simulink model "sensor_simulation"  (R2018a)
settings: Solver=VariableStepAuto  StartTime=0.0  StopTime=10.0  RelTol=1e-3
libraries: simulink x16
(part 1 of 2)
settings Model: Creator=vsbdh  LastModifiedBy=vsbdh

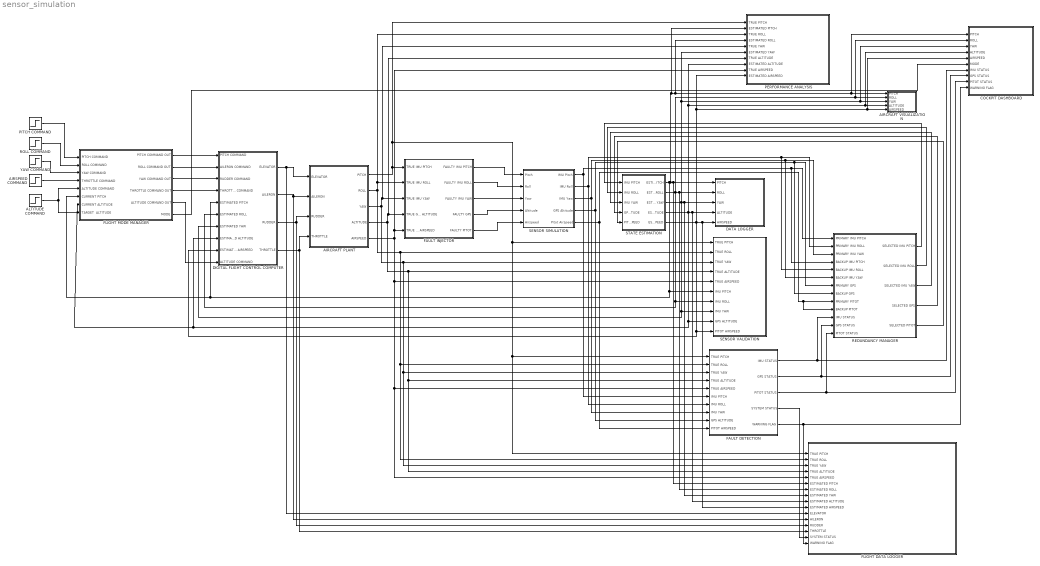
== system sensor_simulation ==
  " SENSOR VALIDATION" : Subsystem
  AIRCRAFT PLANT : Subsystem
  AIRCRAFT VISUALIZATION : Subsystem
  AIRSPEED COMMAND : Step  Time=0  SampleTime=0
  ALTITUDE COMMAND : Step  Time=2  After=1000  SampleTime=0
  COCKPIT DASHBOARD : Subsystem
  DATA LOGGER : Subsystem
  DIGITAL FLIGHT CONTROL COMPUTER : Subsystem
  FAULT DETECTION : Subsystem
  "FAULT INJECTOR " : Subsystem
  FLIGHT DATA LOGGER : Subsystem
  FLIGHT MODE MANAGER : Subsystem
  PERFORMANCE ANALYSIS : Subsystem
  PITCH COMMAND : Step  Time=0  SampleTime=0
  REDUNDANCY MANAGER : Subsystem
  ROLL COMMAND : Step  Time=0  SampleTime=0
  SENSOR SIMULATION : Subsystem
  STATE ESTIMATION : Subsystem
  YAW COMMAND : Step  Time=0  SampleTime=0
  wires:
  AIRCRAFT PLANT/1(PITCH) -> "FAULT INJECTOR "/1(TRUE IMU PITCH), PERFORMANCE ANALYSIS/1(TRUE PITCH), FLIGHT DATA LOGGER/1(TRUE PITCH), FAULT DETECTION/1(TRUE PITCH), " SENSOR VALIDATION"/1(TRUE PITCH)
  AIRCRAFT PLANT/2(ROLL) -> PERFORMANCE ANALYSIS/3(TRUE ROLL), "FAULT INJECTOR "/2(TRUE IMU ROLL), " SENSOR VALIDATION"/2(TRUE ROLL), FAULT DETECTION/2(TRUE ROLL), FLIGHT DATA LOGGER/2(TRUE ROLL)
  AIRCRAFT PLANT/3(YAW) -> PERFORMANCE ANALYSIS/5(TRUE YAW), "FAULT INJECTOR "/3(TRUE IMU YAW), FLIGHT DATA LOGGER/3(TRUE YAW), FAULT DETECTION/3(TRUE YAW), " SENSOR VALIDATION"/3(TRUE YAW)
  AIRCRAFT PLANT/4(ALTITUDE) -> FAULT DETECTION/4(TRUE ALTITUDE), FLIGHT DATA LOGGER/4(TRUE ALTITUDE), " SENSOR VALIDATION"/4(TRUE ALTITUDE), PERFORMANCE ANALYSIS/7(TRUE ALTITUDE), "FAULT INJECTOR "/4(TRUE GPS ALTITUDE)
  AIRCRAFT PLANT/5(AIRSPEED) -> PERFORMANCE ANALYSIS/9(TRUE AIRSPEED), "FAULT INJECTOR "/5(TRUE PITOT AIRSPEED), " SENSOR VALIDATION"/5(TRUE AIRSPEED), FAULT DETECTION/5(TRUE AIRSPEED), FLIGHT DATA LOGGER/5(TRUE AIRSPEED)
  SENSOR SIMULATION/1(IMU Pitch) -> FAULT DETECTION/6(IMU PITCH), REDUNDANCY MANAGER/1(PRIMARY IMU PITCH), REDUNDANCY MANAGER/4(BACKUP IMU PITCH)
  SENSOR SIMULATION/2(IMU Roll) -> FAULT DETECTION/7(IMU ROLL), REDUNDANCY MANAGER/5(BACKUP IMU ROLL), REDUNDANCY MANAGER/2(PRIMARY IMU ROLL)
  SENSOR SIMULATION/3(IMU Yaw) -> FAULT DETECTION/8(IMU YAW), REDUNDANCY MANAGER/6(BACKUP IMU YAW), REDUNDANCY MANAGER/3(PRIMARY IMU YAW)
  SENSOR SIMULATION/4(GPS Altitude) -> FAULT DETECTION/9(GPS ALTITUDE), REDUNDANCY MANAGER/8(BACKUP GPS), REDUNDANCY MANAGER/7(PRIMARY GPS)
  SENSOR SIMULATION/5(Pitot Airspeed) -> FAULT DETECTION/10(PITOT AIRSPEED), REDUNDANCY MANAGER/10(BACKUP PITOT), REDUNDANCY MANAGER/9(PRIMARY PITOT)
  STATE ESTIMATION/1(ESTIMATED PITCH) -> PERFORMANCE ANALYSIS/2(ESTIMATED PITCH), PERFORMANCE ANALYSIS/4(ESTIMATED ROLL), COCKPIT DASHBOARD/1(PITCH), AIRCRAFT VISUALIZATION/1(PITCH), DATA LOGGER/1(PITCH), FLIGHT DATA LOGGER/6(ESTIMATED PITCH), FLIGHT MODE MANAGER/6(CURRENT PITCH), DIGITAL FLIGHT CONTROL COMPUTER/5(ESTIMATED PITCH), " SENSOR VALIDATION"/6(IMU PITCH)
  STATE ESTIMATION/2(ESTIMATED ROLL) -> DIGITAL FLIGHT CONTROL COMPUTER/6(ESTIMATED ROLL), " SENSOR VALIDATION"/7(IMU ROLL), COCKPIT DASHBOARD/2(ROLL), AIRCRAFT VISUALIZATION/2(ROLL), FLIGHT DATA LOGGER/7(ESTIMATED ROLL), DATA LOGGER/2(ROLL)
  STATE ESTIMATION/3(ESTIMATED YAW) -> DIGITAL FLIGHT CONTROL COMPUTER/7(ESTIMATED YAW), " SENSOR VALIDATION"/8(IMU YAW), PERFORMANCE ANALYSIS/6(ESTIMATED YAW), COCKPIT DASHBOARD/3(YAW), AIRCRAFT VISUALIZATION/3(YAW), FLIGHT DATA LOGGER/8(ESTIMATED YAW), DATA LOGGER/3(YAW)
  STATE ESTIMATION/4(ESTIMATED ALTITUDE) -> PERFORMANCE ANALYSIS/8(ESTIMATED ALTITUDE), COCKPIT DASHBOARD/4(ALTITUDE), AIRCRAFT VISUALIZATION/4(ALTITUDE), FLIGHT DATA LOGGER/9(ESTIMATED ALTITUDE), DATA LOGGER/4(ALTITUDE), DIGITAL FLIGHT CONTROL COMPUTER/8(ESTIMATED ALTITUDE), FLIGHT MODE MANAGER/7(CURRENT ALTITUDE), " SENSOR VALIDATION"/9(GPS ALTITUDE)
  STATE ESTIMATION/5(ESTIMATED AIRSPEED) -> PERFORMANCE ANALYSIS/10(ESTIMATED AIRSPEED), COCKPIT DASHBOARD/5(AIRSPEED), AIRCRAFT VISUALIZATION/5(AIRSPEED), FLIGHT DATA LOGGER/10(ESTIMATED AIRSPEED), DATA LOGGER/5(AIRSPEED), DIGITAL FLIGHT CONTROL COMPUTER/9(ESTIMATED AIRSPEED), " SENSOR VALIDATION"/10(PITOT AIRSPEED)
  DIGITAL FLIGHT CONTROL COMPUTER/1(ELEVATOR) -> FLIGHT DATA LOGGER/11(ELEVATOR), AIRCRAFT PLANT/1(ELEVATOR)
  DIGITAL FLIGHT CONTROL COMPUTER/2(AILERON) -> FLIGHT DATA LOGGER/12(AILERON), AIRCRAFT PLANT/2(AILERON)
  DIGITAL FLIGHT CONTROL COMPUTER/3(RUDDER) -> FLIGHT DATA LOGGER/13(RUDDER), AIRCRAFT PLANT/3(RUDDER)
  DIGITAL FLIGHT CONTROL COMPUTER/4(THROTTLE) -> FLIGHT DATA LOGGER/14(THROTTLE), AIRCRAFT PLANT/4(THROTTLE)
  ALTITUDE COMMAND/1 -> FLIGHT MODE MANAGER/8(TARGET  ALTITUDE), FLIGHT MODE MANAGER/5(ALTITUDE COMMAND)
  PITCH COMMAND/1 -> FLIGHT MODE MANAGER/1(PITCH COMMAND)
  ROLL COMMAND/1 -> FLIGHT MODE MANAGER/2(ROLL COMMAND)
  YAW COMMAND/1 -> FLIGHT MODE MANAGER/3(YAW COMMAND)
  AIRSPEED COMMAND/1 -> FLIGHT MODE MANAGER/4(THROTTLE COMMAND)
  FLIGHT MODE MANAGER/1(PITCH COMMAND OUT) -> DIGITAL FLIGHT CONTROL COMPUTER/1(PITCH COMMAND)
  FLIGHT MODE MANAGER/2(ROLL COMMAND OUT) -> DIGITAL FLIGHT CONTROL COMPUTER/2(AILERON COMMAND)
  FLIGHT MODE MANAGER/3(YAW COMMAND OUT) -> DIGITAL FLIGHT CONTROL COMPUTER/3(RUDDER COMMAND)
  FLIGHT MODE MANAGER/4(THROTTLE COMMAND OUT) -> DIGITAL FLIGHT CONTROL COMPUTER/4(THROTTLE COMMAND)
  FLIGHT MODE MANAGER/5(ALTITUDE COMMAND OUT) -> DIGITAL FLIGHT CONTROL COMPUTER/10(ALTITUDE COMMAND)
  FAULT DETECTION/4(SYSTEM STATUS) -> FLIGHT DATA LOGGER/15(SYSTEM STATUS)
  FAULT DETECTION/5(WARNING FLAG) -> FLIGHT DATA LOGGER/16(WARNING FLAG), COCKPIT DASHBOARD/10(WARNING FLAG)
  FAULT DETECTION/1(IMU STATUS) -> COCKPIT DASHBOARD/7(IMU STATUS), REDUNDANCY MANAGER/11(IMU STATUS)
  FAULT DETECTION/2(GPS STATUS) -> COCKPIT DASHBOARD/8(GPS STATUS), REDUNDANCY MANAGER/12(GPS STATUS)
  FAULT DETECTION/3(PITOT STATUS) -> COCKPIT DASHBOARD/9(PITOT STATUS), REDUNDANCY MANAGER/13(PITOT STATUS)
  REDUNDANCY MANAGER/1(SELECTED IMU PITCH) -> STATE ESTIMATION/1(IMU PITCH)
  REDUNDANCY MANAGER/2(SELECTED IMU ROLL) -> STATE ESTIMATION/2(IMU ROLL)
  REDUNDANCY MANAGER/3(SELECTED IMU YAW) -> STATE ESTIMATION/3(IMU YAW)
  REDUNDANCY MANAGER/4(SELECTED GPS) -> STATE ESTIMATION/4(GPS ALTITUDE)
  REDUNDANCY MANAGER/5(SELECTED PITOT) -> STATE ESTIMATION/5(PITOT AIRSPEED)
  "FAULT INJECTOR "/1(FAULTY IMU PITCH) -> SENSOR SIMULATION/1(Pitch)
  "FAULT INJECTOR "/2(FAULTY IMU ROLL) -> SENSOR SIMULATION/2(Roll)
  "FAULT INJECTOR "/3(FAULTY IMU YAW) -> SENSOR SIMULATION/3(Yaw)
  "FAULT INJECTOR "/4(FAULTY GPS) -> SENSOR SIMULATION/4(Altitude)
  "FAULT INJECTOR "/5(FAULTY PITOT) -> SENSOR SIMULATION/5(Airspeed)
  FLIGHT MODE MANAGER/6(MODE) -> COCKPIT DASHBOARD/6(MODE)

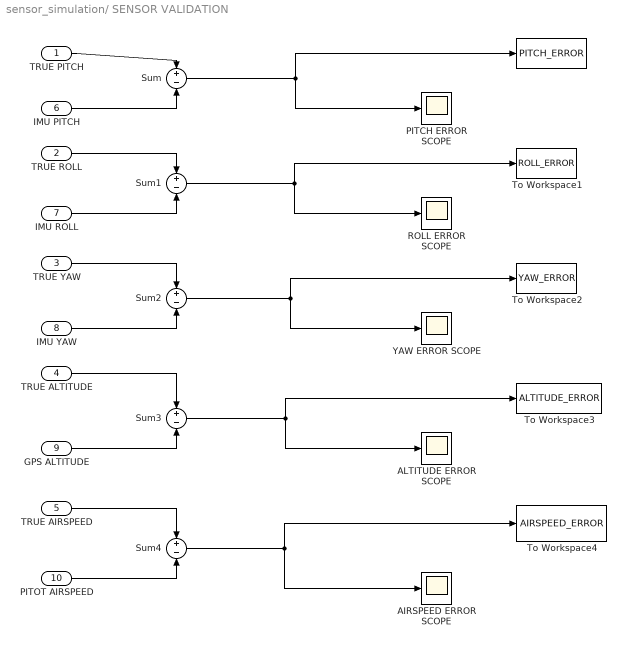
== system sensor_simulation/ SENSOR VALIDATION ==
  TRUE PITCH : Inport
  TRUE ROLL : Inport  Port=2
  TRUE YAW : Inport  Port=3
  TRUE ALTITUDE : Inport  Port=4
  TRUE AIRSPEED : Inport  Port=5
  IMU PITCH : Inport  Port=6
  IMU ROLL : Inport  Port=7
  IMU YAW : Inport  Port=8
  GPS ALTITUDE : Inport  Port=9
  PITOT AIRSPEED : Inport  Port=10
  " " : ToWorkspace  VariableName=PITCH_ERROR  SaveFormat=Structure With Time  SampleTime=-1
  AIRSPEED ERROR SCOPE : Scope
  ALTITUDE ERROR SCOPE : Scope
  PITCH ERROR SCOPE : Scope
  ROLL ERROR SCOPE : Scope
  Sum{,1..4} (5 alike) : Sum  Inputs=+-
  To Workspace1 : ToWorkspace  VariableName=ROLL_ERROR  SaveFormat=Structure With Time  SampleTime=-1
  To Workspace2 : ToWorkspace  VariableName=YAW_ERROR  SaveFormat=Structure With Time  SampleTime=-1
  To Workspace3 : ToWorkspace  VariableName=ALTITUDE_ERROR  SaveFormat=Structure With Time  SampleTime=-1
  To Workspace4 : ToWorkspace  VariableName=AIRSPEED_ERROR  SaveFormat=Structure With Time  SampleTime=-1
  YAW ERROR SCOPE : Scope
  wires:
  TRUE PITCH/1 -> Sum/1
  IMU PITCH/1 -> Sum/2
  Sum/1 -> " "/1, PITCH ERROR SCOPE/1
  TRUE ROLL/1 -> Sum1/1
  IMU ROLL/1 -> Sum1/2
  Sum1/1 -> To Workspace1/1, ROLL ERROR SCOPE/1
  TRUE YAW/1 -> Sum2/1
  IMU YAW/1 -> Sum2/2
  Sum2/1 -> To Workspace2/1, YAW ERROR SCOPE/1
  TRUE ALTITUDE/1 -> Sum3/1
  GPS ALTITUDE/1 -> Sum3/2
  Sum3/1 -> To Workspace3/1, ALTITUDE ERROR SCOPE/1
  TRUE AIRSPEED/1 -> Sum4/1
  PITOT AIRSPEED/1 -> Sum4/2
  Sum4/1 -> AIRSPEED ERROR SCOPE/1, To Workspace4/1

== system sensor_simulation/AIRCRAFT PLANT ==
  ELEVATOR : Inport
  AILERON : Inport  Port=2
  RUDDER : Inport  Port=3
  THROTTLE : Inport  Port=4
  AIRSPEED DYNAMICS : Subsystem
  ALTITUDE DYNAMICS : Subsystem
  PITCH DYNAMICS : Subsystem
  ROLL DYNAMICS : Subsystem
  YAW DYNAMICS : Subsystem
  PITCH : Outport
  ROLL : Outport  Port=2
  YAW : Outport  Port=3
  ALTITUDE : Outport  Port=4
  AIRSPEED : Outport  Port=5
  wires:
  ELEVATOR/1 -> PITCH DYNAMICS/1(ELEVATOR)
  PITCH DYNAMICS/1(PITCH) -> PITCH/1, ALTITUDE DYNAMICS/1(PITCH)
  ALTITUDE DYNAMICS/1(ALTITUDE) -> ALTITUDE/1
  AILERON/1 -> ROLL DYNAMICS/1(AILERON)
  ROLL DYNAMICS/1(ROLL) -> ROLL/1
  RUDDER/1 -> YAW DYNAMICS/1(RUDDER)
  YAW DYNAMICS/1(YAW) -> YAW/1
  THROTTLE/1 -> AIRSPEED DYNAMICS/1("THROTTLE ")
  AIRSPEED DYNAMICS/1(AIRSPEED) -> AIRSPEED/1

== system sensor_simulation/AIRCRAFT VISUALIZATION ==
  PITCH : Inport
  ROLL : Inport  Port=2
  YAW : Inport  Port=3
  ALTITUDE : Inport  Port=4
  AIRSPEED : Inport  Port=5
  AIRSPEED SCOPE : Scope
  ALTITUDE SCOPE : Scope
  PITCH SCOPE : Scope
  ROLL SCOPE : Scope
  YAW SCOPE : Scope
  wires:
  PITCH/1 -> PITCH SCOPE/1
  ROLL/1 -> ROLL SCOPE/1
  YAW/1 -> YAW SCOPE/1
  ALTITUDE/1 -> ALTITUDE SCOPE/1
  AIRSPEED/1 -> AIRSPEED SCOPE/1

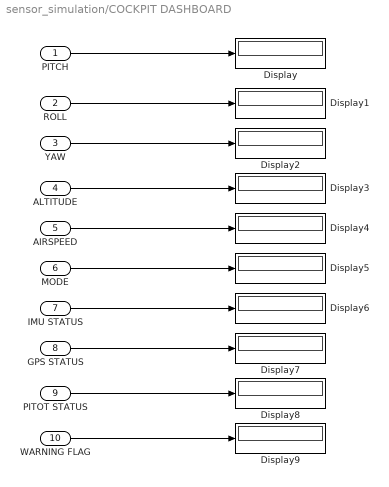
== system sensor_simulation/COCKPIT DASHBOARD ==
  PITCH : Inport
  ROLL : Inport  Port=2
  YAW : Inport  Port=3
  ALTITUDE : Inport  Port=4
  AIRSPEED : Inport  Port=5
  MODE : Inport  Port=6
  IMU STATUS : Inport  Port=7
  GPS STATUS : Inport  Port=8
  PITOT STATUS : Inport  Port=9
  WARNING FLAG : Inport  Port=10
  Display{,1..9} (10 alike) : Display
  wires:
  PITCH/1 -> Display/1
  ROLL/1 -> Display1/1
  YAW/1 -> Display2/1
  ALTITUDE/1 -> Display3/1
  AIRSPEED/1 -> Display4/1
  MODE/1 -> Display5/1
  IMU STATUS/1 -> Display6/1
  GPS STATUS/1 -> Display7/1
  PITOT STATUS/1 -> Display8/1
  WARNING FLAG/1 -> Display9/1

== system sensor_simulation/DATA LOGGER ==
  PITCH : Inport
  ROLL : Inport  Port=2
  YAW : Inport  Port=3
  ALTITUDE : Inport  Port=4
  AIRSPEED : Inport  Port=5
  AIRSPEED DATA : ToWorkspace  VariableName=airspeed_data  SaveFormat=Structure With Time  SampleTime=-1
  ALTITUDE DATA : ToWorkspace  VariableName=altitude_data  SaveFormat=Structure With Time  SampleTime=-1
  PITCH DATA : ToWorkspace  VariableName=pitch_data  SaveFormat=Structure With Time  SampleTime=-1
  ROLL DATA : ToWorkspace  VariableName=roll_data  SaveFormat=Structure With Time  SampleTime=-1
  YAW DATA : ToWorkspace  VariableName=yaw_data  SaveFormat=Structure With Time  SampleTime=-1
  wires:
  PITCH/1 -> PITCH DATA/1
  ROLL/1 -> ROLL DATA/1
  YAW/1 -> YAW DATA/1
  ALTITUDE/1 -> ALTITUDE DATA/1
  AIRSPEED/1 -> AIRSPEED DATA/1

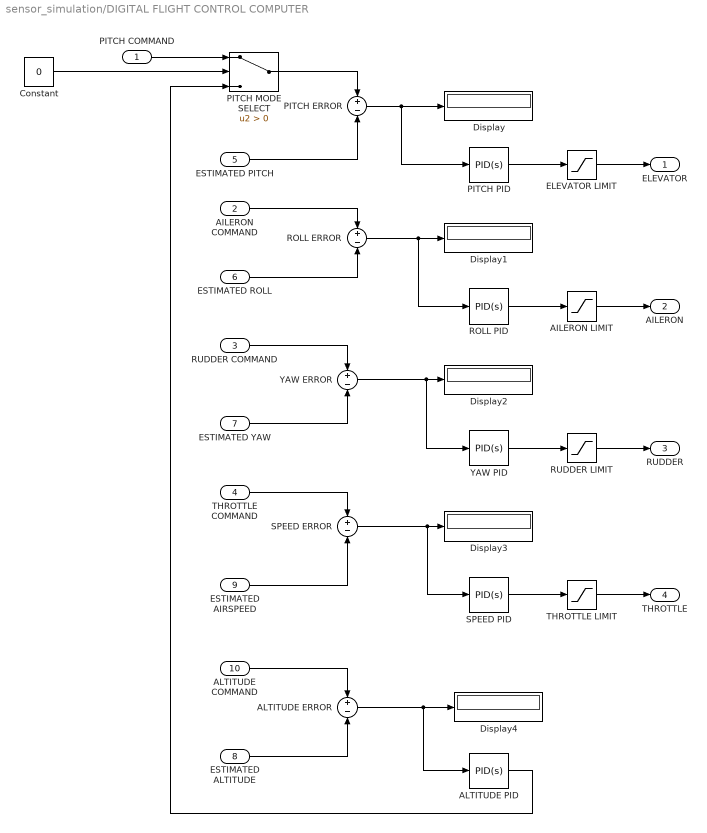
== system sensor_simulation/DIGITAL FLIGHT CONTROL COMPUTER ==
  PITCH COMMAND : Inport
  AILERON COMMAND : Inport  Port=2
  RUDDER COMMAND : Inport  Port=3
  THROTTLE COMMAND : Inport  Port=4
  ESTIMATED PITCH : Inport  Port=5
  ESTIMATED ROLL : Inport  Port=6
  ESTIMATED YAW : Inport  Port=7
  ESTIMATED ALTITUDE : Inport  Port=8
  ESTIMATED AIRSPEED : Inport  Port=9
  ALTITUDE COMMAND : Inport  Port=10
  " ALTITUDE ERROR" : Sum  Inputs=+-
  " PITCH ERROR" : Sum  Inputs=+-
  " ROLL ERROR" : Sum  Inputs=+-
  " SPEED ERROR" : Sum  Inputs=+-
  " YAW ERROR" : Sum  Inputs=+-
  AILERON LIMIT : Saturate  UpperLimit=1  LowerLimit=-1
  ALTITUDE PID : simulink/Continuous/PID Controller  Controller=PID  TimeDomain=Continuous-time  SampleTime=-1  IntegratorMethod=Forward Euler  FilterMethod=Forward Euler  Form=Parallel  UseFilter=on  ControllerParametersSource=internal  P=0.8  I=0.2  D=0  N=100  InitialConditionSource=internal  InitialConditionForIntegrator=0  InitialConditionForFilter=0  ExternalReset=none  LimitOutput=off  UpperSaturationLimit=inf  LowerSaturationLimit=-inf  LinearizeAsGain=on  AntiWindupMode=none  Kb=1  TrackingMode=off  Kt=1  PParamMin=[]  PParamMax=[]  IParamMin=[]  IParamMax=[]  DParamMin=[]  DParamMax=[]  NParamMin=[]  NParamMax=[]  KbParamMin=[]  KbParamMax=[]  KtParamMin=[]  KtParamMax=[]  POutMin=[]  POutMax=[]  IOutMin=[]  IOutMax=[]  DOutMin=[]  DOutMax=[]  NOutMin=[]  NOutMax=[]  KbOutMin=[]  KbOutMax=[]  KtOutMin=[]  KtOutMax=[]  IntegratorOutMin=[]  IntegratorOutMax=[]  FilterOutMin=[]  FilterOutMax=[]  SumOutMin=[]  SumOutMax=[]  SumI1OutMin=[]  SumI1OutMax=[]  SumI2OutMin=[]  SumI2OutMax=[]  SumI3OutMin=[]  SumI3OutMax=[]  SumDOutMin=[]  SumDOutMax=[]  SaturationOutMin=[]  SaturationOutMax=[]  IntegratorContinuousStateAttributes=''  IntegratorStateMustResolveToSignalObject=off  IntegratorRTWStateStorageClass=Auto  FilterContinuousStateAttributes=''  FilterStateMustResolveToSignalObject=off  FilterRTWStateStorageClass=Auto  DifferentiatorICPrevScaledInput=0  DifferentiatorOutMin=[]  DifferentiatorOutMax=[]  FilterDiffOutCoefMin=[]  FilterDiffOutCoefMax=[]  SumDenOutMin=[]  SumDenOutMax=[]  SumNumOutMin=[]  SumNumOutMax=[]  ReciprocalOutMin=[]  ReciprocalOutMax=[]  DivideOutMin=[]  DivideOutMax=[]  TunerSelectOption=Transfer Function Based (PID Tuner App)
  Constant : Constant  Value=0
  Display{,1..4} (5 alike) : Display
  ELEVATOR LIMIT : Saturate  UpperLimit=1  LowerLimit=-1
  PITCH MODE SELECT : Switch  Criteria=u2 > Threshold
  PITCH PID : simulink/Continuous/PID Controller  Controller=PID  TimeDomain=Continuous-time  SampleTime=-1  IntegratorMethod=Forward Euler  FilterMethod=Forward Euler  Form=Parallel  UseFilter=on  ControllerParametersSource=internal  P=2  I=0.5  D=0.1  N=100  InitialConditionSource=internal  InitialConditionForIntegrator=0  InitialConditionForFilter=0  ExternalReset=none  LimitOutput=off  UpperSaturationLimit=inf  LowerSaturationLimit=-inf  LinearizeAsGain=on  AntiWindupMode=none  Kb=1  TrackingMode=off  Kt=1  PParamMin=[]  PParamMax=[]  IParamMin=[]  IParamMax=[]  DParamMin=[]  DParamMax=[]  NParamMin=[]  NParamMax=[]  KbParamMin=[]  KbParamMax=[]  KtParamMin=[]  KtParamMax=[]  POutMin=[]  POutMax=[]  IOutMin=[]  IOutMax=[]  DOutMin=[]  DOutMax=[]  NOutMin=[]  NOutMax=[]  KbOutMin=[]  KbOutMax=[]  KtOutMin=[]  KtOutMax=[]  IntegratorOutMin=[]  IntegratorOutMax=[]  FilterOutMin=[]  FilterOutMax=[]  SumOutMin=[]  SumOutMax=[]  SumI1OutMin=[]  SumI1OutMax=[]  SumI2OutMin=[]  SumI2OutMax=[]  SumI3OutMin=[]  SumI3OutMax=[]  SumDOutMin=[]  SumDOutMax=[]  SaturationOutMin=[]  SaturationOutMax=[]  IntegratorContinuousStateAttributes=''  IntegratorStateMustResolveToSignalObject=off  IntegratorRTWStateStorageClass=Auto  FilterContinuousStateAttributes=''  FilterStateMustResolveToSignalObject=off  FilterRTWStateStorageClass=Auto  DifferentiatorICPrevScaledInput=0  DifferentiatorOutMin=[]  DifferentiatorOutMax=[]  FilterDiffOutCoefMin=[]  FilterDiffOutCoefMax=[]  SumDenOutMin=[]  SumDenOutMax=[]  SumNumOutMin=[]  SumNumOutMax=[]  ReciprocalOutMin=[]  ReciprocalOutMax=[]  DivideOutMin=[]  DivideOutMax=[]  TunerSelectOption=Transfer Function Based (PID Tuner App)
  ROLL PID : simulink/Continuous/PID Controller  Controller=PID  TimeDomain=Continuous-time  SampleTime=-1  IntegratorMethod=Forward Euler  FilterMethod=Forward Euler  Form=Parallel  UseFilter=on  ControllerParametersSource=internal  P=2  I=0.5  D=0.1  N=100  InitialConditionSource=internal  InitialConditionForIntegrator=0  InitialConditionForFilter=0  ExternalReset=none  LimitOutput=off  UpperSaturationLimit=inf  LowerSaturationLimit=-inf  LinearizeAsGain=on  AntiWindupMode=none  Kb=1  TrackingMode=off  Kt=1  PParamMin=[]  PParamMax=[]  IParamMin=[]  IParamMax=[]  DParamMin=[]  DParamMax=[]  NParamMin=[]  NParamMax=[]  KbParamMin=[]  KbParamMax=[]  KtParamMin=[]  KtParamMax=[]  POutMin=[]  POutMax=[]  IOutMin=[]  IOutMax=[]  DOutMin=[]  DOutMax=[]  NOutMin=[]  NOutMax=[]  KbOutMin=[]  KbOutMax=[]  KtOutMin=[]  KtOutMax=[]  IntegratorOutMin=[]  IntegratorOutMax=[]  FilterOutMin=[]  FilterOutMax=[]  SumOutMin=[]  SumOutMax=[]  SumI1OutMin=[]  SumI1OutMax=[]  SumI2OutMin=[]  SumI2OutMax=[]  SumI3OutMin=[]  SumI3OutMax=[]  SumDOutMin=[]  SumDOutMax=[]  SaturationOutMin=[]  SaturationOutMax=[]  IntegratorContinuousStateAttributes=''  IntegratorStateMustResolveToSignalObject=off  IntegratorRTWStateStorageClass=Auto  FilterContinuousStateAttributes=''  FilterStateMustResolveToSignalObject=off  FilterRTWStateStorageClass=Auto  DifferentiatorICPrevScaledInput=0  DifferentiatorOutMin=[]  DifferentiatorOutMax=[]  FilterDiffOutCoefMin=[]  FilterDiffOutCoefMax=[]  SumDenOutMin=[]  SumDenOutMax=[]  SumNumOutMin=[]  SumNumOutMax=[]  ReciprocalOutMin=[]  ReciprocalOutMax=[]  DivideOutMin=[]  DivideOutMax=[]  TunerSelectOption=Transfer Function Based (PID Tuner App)
  RUDDER LIMIT : Saturate  UpperLimit=1  LowerLimit=-1
  SPEED PID : simulink/Continuous/PID Controller  Controller=PID  TimeDomain=Continuous-time  SampleTime=-1  IntegratorMethod=Forward Euler  FilterMethod=Forward Euler  Form=Parallel  UseFilter=on  ControllerParametersSource=internal  P=2  I=0.5  D=0.1  N=100  InitialConditionSource=internal  InitialConditionForIntegrator=0  InitialConditionForFilter=0  ExternalReset=none  LimitOutput=off  UpperSaturationLimit=inf  LowerSaturationLimit=-inf  LinearizeAsGain=on  AntiWindupMode=none  Kb=1  TrackingMode=off  Kt=1  PParamMin=[]  PParamMax=[]  IParamMin=[]  IParamMax=[]  DParamMin=[]  DParamMax=[]  NParamMin=[]  NParamMax=[]  KbParamMin=[]  KbParamMax=[]  KtParamMin=[]  KtParamMax=[]  POutMin=[]  POutMax=[]  IOutMin=[]  IOutMax=[]  DOutMin=[]  DOutMax=[]  NOutMin=[]  NOutMax=[]  KbOutMin=[]  KbOutMax=[]  KtOutMin=[]  KtOutMax=[]  IntegratorOutMin=[]  IntegratorOutMax=[]  FilterOutMin=[]  FilterOutMax=[]  SumOutMin=[]  SumOutMax=[]  SumI1OutMin=[]  SumI1OutMax=[]  SumI2OutMin=[]  SumI2OutMax=[]  SumI3OutMin=[]  SumI3OutMax=[]  SumDOutMin=[]  SumDOutMax=[]  SaturationOutMin=[]  SaturationOutMax=[]  IntegratorContinuousStateAttributes=''  IntegratorStateMustResolveToSignalObject=off  IntegratorRTWStateStorageClass=Auto  FilterContinuousStateAttributes=''  FilterStateMustResolveToSignalObject=off  FilterRTWStateStorageClass=Auto  DifferentiatorICPrevScaledInput=0  DifferentiatorOutMin=[]  DifferentiatorOutMax=[]  FilterDiffOutCoefMin=[]  FilterDiffOutCoefMax=[]  SumDenOutMin=[]  SumDenOutMax=[]  SumNumOutMin=[]  SumNumOutMax=[]  ReciprocalOutMin=[]  ReciprocalOutMax=[]  DivideOutMin=[]  DivideOutMax=[]  TunerSelectOption=Transfer Function Based (PID Tuner App)
  THROTTLE LIMIT : Saturate  UpperLimit=1  LowerLimit=0
  YAW PID : simulink/Continuous/PID Controller  Controller=PID  TimeDomain=Continuous-time  SampleTime=-1  IntegratorMethod=Forward Euler  FilterMethod=Forward Euler  Form=Parallel  UseFilter=on  ControllerParametersSource=internal  P=2  I=0.5  D=0.1  N=100  InitialConditionSource=internal  InitialConditionForIntegrator=0  InitialConditionForFilter=0  ExternalReset=none  LimitOutput=off  UpperSaturationLimit=inf  LowerSaturationLimit=-inf  LinearizeAsGain=on  AntiWindupMode=none  Kb=1  TrackingMode=off  Kt=1  PParamMin=[]  PParamMax=[]  IParamMin=[]  IParamMax=[]  DParamMin=[]  DParamMax=[]  NParamMin=[]  NParamMax=[]  KbParamMin=[]  KbParamMax=[]  KtParamMin=[]  KtParamMax=[]  POutMin=[]  POutMax=[]  IOutMin=[]  IOutMax=[]  DOutMin=[]  DOutMax=[]  NOutMin=[]  NOutMax=[]  KbOutMin=[]  KbOutMax=[]  KtOutMin=[]  KtOutMax=[]  IntegratorOutMin=[]  IntegratorOutMax=[]  FilterOutMin=[]  FilterOutMax=[]  SumOutMin=[]  SumOutMax=[]  SumI1OutMin=[]  SumI1OutMax=[]  SumI2OutMin=[]  SumI2OutMax=[]  SumI3OutMin=[]  SumI3OutMax=[]  SumDOutMin=[]  SumDOutMax=[]  SaturationOutMin=[]  SaturationOutMax=[]  IntegratorContinuousStateAttributes=''  IntegratorStateMustResolveToSignalObject=off  IntegratorRTWStateStorageClass=Auto  FilterContinuousStateAttributes=''  FilterStateMustResolveToSignalObject=off  FilterRTWStateStorageClass=Auto  DifferentiatorICPrevScaledInput=0  DifferentiatorOutMin=[]  DifferentiatorOutMax=[]  FilterDiffOutCoefMin=[]  FilterDiffOutCoefMax=[]  SumDenOutMin=[]  SumDenOutMax=[]  SumNumOutMin=[]  SumNumOutMax=[]  ReciprocalOutMin=[]  ReciprocalOutMax=[]  DivideOutMin=[]  DivideOutMax=[]  TunerSelectOption=Transfer Function Based (PID Tuner App)
  ELEVATOR : Outport
  AILERON : Outport  Port=2
  RUDDER : Outport  Port=3
  THROTTLE : Outport  Port=4
  wires:
  ESTIMATED PITCH/1 -> " PITCH ERROR"/2
  AILERON COMMAND/1 -> " ROLL ERROR"/1
  ESTIMATED ROLL/1 -> " ROLL ERROR"/2
  RUDDER COMMAND/1 -> " YAW ERROR"/1
  ESTIMATED YAW/1 -> " YAW ERROR"/2
  THROTTLE COMMAND/1 -> " SPEED ERROR"/1
  ESTIMATED AIRSPEED/1 -> " SPEED ERROR"/2
  " PITCH ERROR"/1 -> PITCH PID/1, Display/1
  " ROLL ERROR"/1 -> ROLL PID/1, Display1/1
  " YAW ERROR"/1 -> YAW PID/1, Display2/1
  " SPEED ERROR"/1 -> SPEED PID/1, Display3/1
  PITCH PID/1 -> ELEVATOR LIMIT/1
  ELEVATOR LIMIT/1 -> ELEVATOR/1
  ROLL PID/1 -> AILERON LIMIT/1
  AILERON LIMIT/1 -> AILERON/1
  YAW PID/1 -> RUDDER LIMIT/1
  RUDDER LIMIT/1 -> RUDDER/1
  SPEED PID/1 -> THROTTLE LIMIT/1
  THROTTLE LIMIT/1 -> THROTTLE/1
  ALTITUDE COMMAND/1 -> " ALTITUDE ERROR"/1
  ESTIMATED ALTITUDE/1 -> " ALTITUDE ERROR"/2
  " ALTITUDE ERROR"/1 -> ALTITUDE PID/1, Display4/1
  PITCH COMMAND/1 -> PITCH MODE SELECT/1
  ALTITUDE PID/1 -> PITCH MODE SELECT/3
  Constant/1 -> PITCH MODE SELECT/2
  PITCH MODE SELECT/1 -> " PITCH ERROR"/1

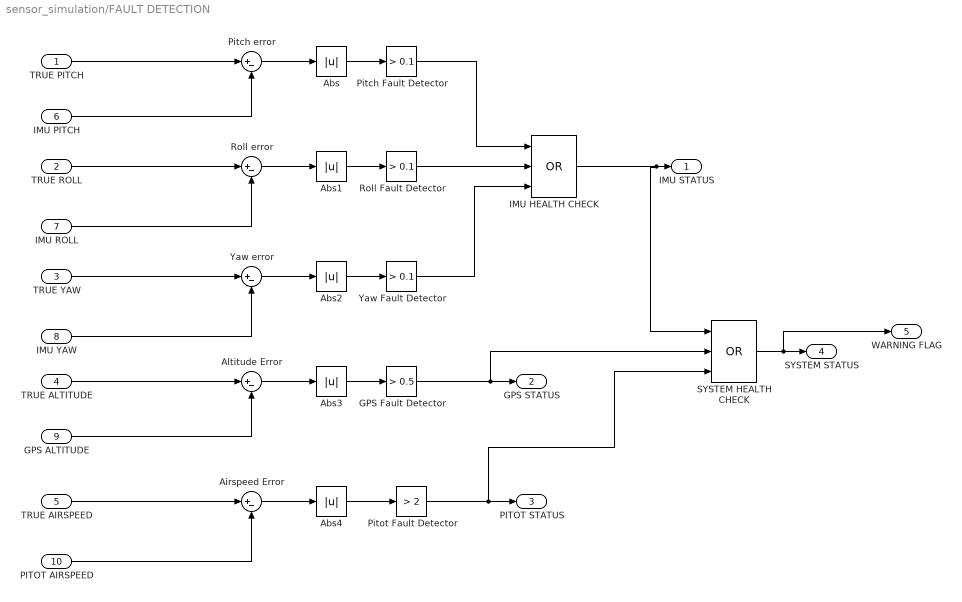
== system sensor_simulation/FAULT DETECTION ==
  TRUE PITCH : Inport
  TRUE ROLL : Inport  Port=2
  TRUE YAW : Inport  Port=3
  TRUE ALTITUDE : Inport  Port=4
  TRUE AIRSPEED : Inport  Port=5
  IMU PITCH : Inport  Port=6
  IMU ROLL : Inport  Port=7
  IMU YAW : Inport  Port=8
  GPS ALTITUDE : Inport  Port=9
  PITOT AIRSPEED : Inport  Port=10
  " Airspeed Error" : Sum  Inputs=|+-
  " Altitude Error" : Sum  Inputs=|+-
  " Pitch error" : Sum  Inputs=|+-
  " Roll error" : Sum  Inputs=|+-
  " Yaw error" : Sum  Inputs=|+-
  Abs{,1..4} (5 alike) : Abs
  GPS Fault Detector : simulink/Logic and Bit Operations/Compare To Constant  relop=>  const=0.5  OutDataTypeStr=boolean
  IMU HEALTH CHECK : Logic  Operator=OR  Inputs=3  AllPortsSameDT=off  OutDataTypeStr=boolean
  Pitch Fault Detector : simulink/Logic and Bit Operations/Compare To Constant  relop=>  const=0.1  OutDataTypeStr=boolean
  Pitot Fault Detector : simulink/Logic and Bit Operations/Compare To Constant  relop=>  const=2  OutDataTypeStr=boolean
  Roll Fault Detector : simulink/Logic and Bit Operations/Compare To Constant  relop=>  const=0.1  OutDataTypeStr=boolean
  SYSTEM HEALTH CHECK : Logic  Operator=OR  Inputs=3  AllPortsSameDT=off  OutDataTypeStr=boolean
  Yaw Fault Detector : simulink/Logic and Bit Operations/Compare To Constant  relop=>  const=0.1  OutDataTypeStr=boolean
  IMU STATUS : Outport
  GPS STATUS : Outport  Port=2
  PITOT STATUS : Outport  Port=3
  SYSTEM STATUS : Outport  Port=4
  WARNING FLAG : Outport  Port=5
  wires:
  TRUE PITCH/1 -> " Pitch error"/1
  IMU PITCH/1 -> " Pitch error"/2
  TRUE ROLL/1 -> " Roll error"/1
  IMU ROLL/1 -> " Roll error"/2
  " Pitch error"/1 -> Abs/1
  Abs/1 -> Pitch Fault Detector/1
  " Roll error"/1 -> Abs1/1
  Abs1/1 -> Roll Fault Detector/1
  TRUE YAW/1 -> " Yaw error"/1
  IMU YAW/1 -> " Yaw error"/2
  " Yaw error"/1 -> Abs2/1
  Abs2/1 -> Yaw Fault Detector/1
  Roll Fault Detector/1 -> IMU HEALTH CHECK/2
  Pitch Fault Detector/1 -> IMU HEALTH CHECK/1
  Yaw Fault Detector/1 -> IMU HEALTH CHECK/3
  IMU HEALTH CHECK/1 -> SYSTEM HEALTH CHECK/1, IMU STATUS/1
  " Altitude Error"/1 -> Abs3/1
  TRUE ALTITUDE/1 -> " Altitude Error"/1
  GPS ALTITUDE/1 -> " Altitude Error"/2
  Abs3/1 -> GPS Fault Detector/1
  GPS Fault Detector/1 -> SYSTEM HEALTH CHECK/2, GPS STATUS/1
  TRUE AIRSPEED/1 -> " Airspeed Error"/1
  PITOT AIRSPEED/1 -> " Airspeed Error"/2
  " Airspeed Error"/1 -> Abs4/1
  Abs4/1 -> Pitot Fault Detector/1
  Pitot Fault Detector/1 -> SYSTEM HEALTH CHECK/3, PITOT STATUS/1
  SYSTEM HEALTH CHECK/1 -> WARNING FLAG/1, SYSTEM STATUS/1

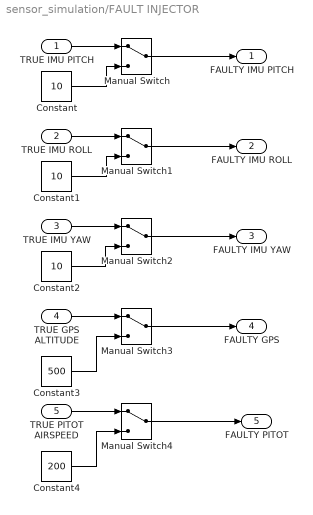
== system sensor_simulation/FAULT INJECTOR  ==
  TRUE IMU PITCH : Inport
  TRUE IMU ROLL : Inport  Port=2
  TRUE IMU YAW : Inport  Port=3
  TRUE GPS ALTITUDE : Inport  Port=4
  TRUE PITOT AIRSPEED : Inport  Port=5
  Constant : Constant  Value=10
  Constant1 : Constant  Value=10
  Constant2 : Constant  Value=10
  Constant3 : Constant  Value=500
  Constant4 : Constant  Value=200
  Manual Switch{,1..4} (5 alike) : ManualSwitch
  FAULTY IMU PITCH : Outport
  FAULTY IMU ROLL : Outport  Port=2
  FAULTY IMU YAW : Outport  Port=3
  FAULTY GPS : Outport  Port=4
  FAULTY PITOT : Outport  Port=5
  wires:
  TRUE IMU PITCH/1 -> Manual Switch/1
  Constant/1 -> Manual Switch/2
  Manual Switch/1 -> FAULTY IMU PITCH/1
  TRUE IMU ROLL/1 -> Manual Switch1/1
  Manual Switch1/1 -> FAULTY IMU ROLL/1
  Constant1/1 -> Manual Switch1/2
  TRUE IMU YAW/1 -> Manual Switch2/1
  Manual Switch2/1 -> FAULTY IMU YAW/1
  Constant2/1 -> Manual Switch2/2
  TRUE GPS ALTITUDE/1 -> Manual Switch3/1
  Constant3/1 -> Manual Switch3/2
  Manual Switch3/1 -> FAULTY GPS/1
  TRUE PITOT AIRSPEED/1 -> Manual Switch4/1
  Manual Switch4/1 -> FAULTY PITOT/1
  Constant4/1 -> Manual Switch4/2

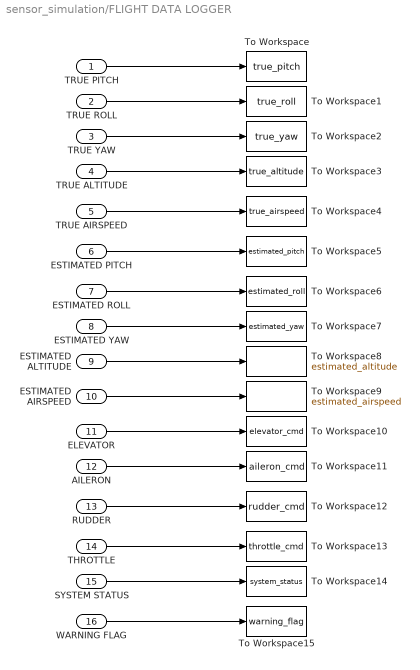
== system sensor_simulation/FLIGHT DATA LOGGER ==
  TRUE PITCH : Inport
  TRUE ROLL : Inport  Port=2
  TRUE YAW : Inport  Port=3
  TRUE ALTITUDE : Inport  Port=4
  TRUE AIRSPEED : Inport  Port=5
  ESTIMATED PITCH : Inport  Port=6
  ESTIMATED ROLL : Inport  Port=7
  ESTIMATED YAW : Inport  Port=8
  ESTIMATED ALTITUDE : Inport  Port=9
  ESTIMATED AIRSPEED : Inport  Port=10
  ELEVATOR : Inport  Port=11
  AILERON : Inport  Port=12
  RUDDER : Inport  Port=13
  THROTTLE : Inport  Port=14
  SYSTEM STATUS : Inport  Port=15
  WARNING FLAG : Inport  Port=16
  To Workspace : ToWorkspace  VariableName=true_pitch  SampleTime=-1
  To Workspace1 : ToWorkspace  VariableName=true_roll  SampleTime=-1
  To Workspace10 : ToWorkspace  VariableName=elevator_cmd  SampleTime=-1
  To Workspace11 : ToWorkspace  VariableName=aileron_cmd  SampleTime=-1
  To Workspace12 : ToWorkspace  VariableName=rudder_cmd  SampleTime=-1
  To Workspace13 : ToWorkspace  VariableName=throttle_cmd  SampleTime=-1
  To Workspace14 : ToWorkspace  VariableName=system_status  SampleTime=-1
  To Workspace15 : ToWorkspace  VariableName=warning_flag  SampleTime=-1
  To Workspace2 : ToWorkspace  VariableName=true_yaw  SampleTime=-1
  To Workspace3 : ToWorkspace  VariableName=true_altitude  SampleTime=-1
  To Workspace4 : ToWorkspace  VariableName=true_airspeed  SampleTime=-1
  To Workspace5 : ToWorkspace  VariableName=estimated_pitch  SampleTime=-1
  To Workspace6 : ToWorkspace  VariableName=estimated_roll  SampleTime=-1
  To Workspace7 : ToWorkspace  VariableName=estimated_yaw  SampleTime=-1
  To Workspace8 : ToWorkspace  VariableName=estimated_altitude  SampleTime=-1
  To Workspace9 : ToWorkspace  VariableName=estimated_airspeed  SampleTime=-1
  wires:
  TRUE PITCH/1 -> To Workspace/1
  TRUE ROLL/1 -> To Workspace1/1
  TRUE YAW/1 -> To Workspace2/1
  TRUE ALTITUDE/1 -> To Workspace3/1
  TRUE AIRSPEED/1 -> To Workspace4/1
  ESTIMATED PITCH/1 -> To Workspace5/1
  ESTIMATED ROLL/1 -> To Workspace6/1
  ESTIMATED YAW/1 -> To Workspace7/1
  ESTIMATED ALTITUDE/1 -> To Workspace8/1
  ESTIMATED AIRSPEED/1 -> To Workspace9/1
  ELEVATOR/1 -> To Workspace10/1
  AILERON/1 -> To Workspace11/1
  RUDDER/1 -> To Workspace12/1
  THROTTLE/1 -> To Workspace13/1
  SYSTEM STATUS/1 -> To Workspace14/1
  WARNING FLAG/1 -> To Workspace15/1

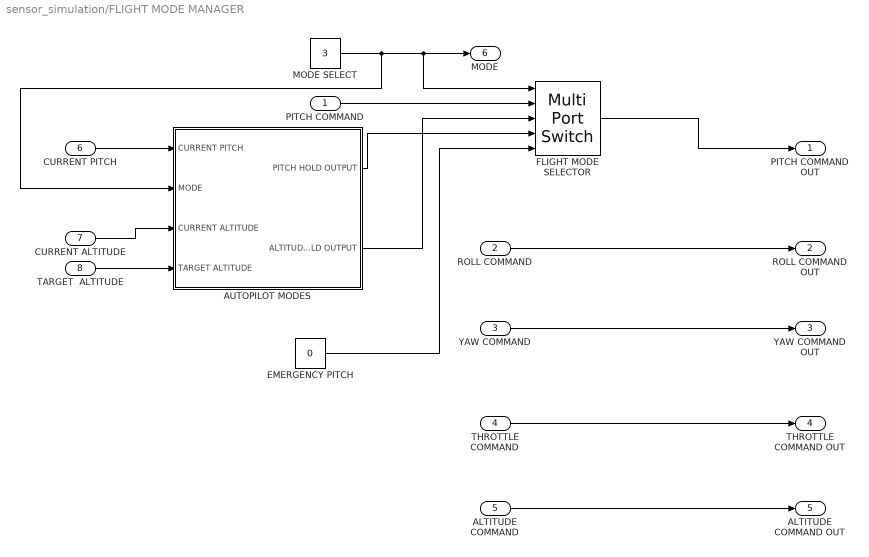
== system sensor_simulation/FLIGHT MODE MANAGER ==
  PITCH COMMAND : Inport
  ROLL COMMAND : Inport  Port=2
  YAW COMMAND : Inport  Port=3
  THROTTLE COMMAND : Inport  Port=4
  ALTITUDE COMMAND : Inport  Port=5
  CURRENT PITCH : Inport  Port=6
  CURRENT ALTITUDE : Inport  Port=7
  TARGET  ALTITUDE : Inport  Port=8
  AUTOPILOT MODES : Subsystem
  EMERGENCY PITCH : Constant  Value=0
  "FLIGHT MODE SELECTOR " : MultiPortSwitch  Inputs=4
  MODE SELECT : Constant  Value=3
  PITCH COMMAND OUT : Outport
  ROLL COMMAND OUT : Outport  Port=2
  YAW COMMAND OUT : Outport  Port=3
  THROTTLE COMMAND OUT : Outport  Port=4
  ALTITUDE COMMAND OUT : Outport  Port=5
  MODE : Outport  Port=6
  wires:
  ROLL COMMAND/1 -> ROLL COMMAND OUT/1
  YAW COMMAND/1 -> YAW COMMAND OUT/1
  THROTTLE COMMAND/1 -> THROTTLE COMMAND OUT/1
  PITCH COMMAND/1 -> "FLIGHT MODE SELECTOR "/2
  ALTITUDE COMMAND/1 -> ALTITUDE COMMAND OUT/1
  MODE SELECT/1 -> MODE/1, "FLIGHT MODE SELECTOR "/1, AUTOPILOT MODES/2(MODE)
  EMERGENCY PITCH/1 -> "FLIGHT MODE SELECTOR "/5
  "FLIGHT MODE SELECTOR "/1 -> PITCH COMMAND OUT/1
  AUTOPILOT MODES/1(PITCH HOLD OUTPUT) -> "FLIGHT MODE SELECTOR "/4
  AUTOPILOT MODES/2(ALTITUDE HOLD OUTPUT) -> "FLIGHT MODE SELECTOR "/3
  CURRENT PITCH/1 -> AUTOPILOT MODES/1(CURRENT PITCH)
  CURRENT ALTITUDE/1 -> AUTOPILOT MODES/3(CURRENT ALTITUDE)
  TARGET  ALTITUDE/1 -> AUTOPILOT MODES/4(TARGET ALTITUDE)

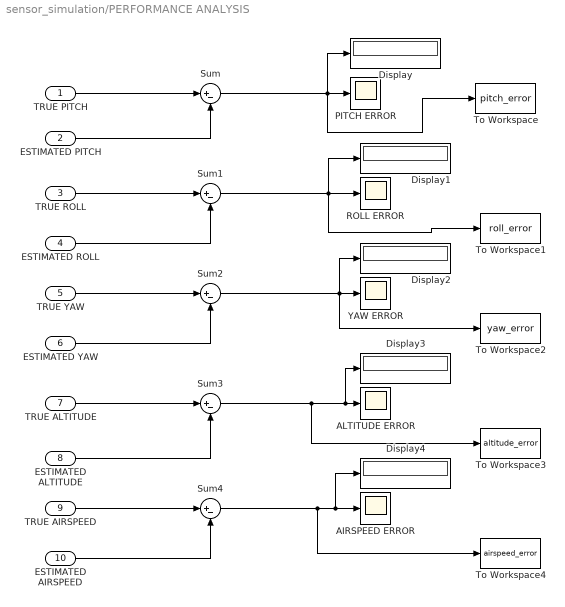
== system sensor_simulation/PERFORMANCE ANALYSIS ==
  TRUE PITCH : Inport
  ESTIMATED PITCH : Inport  Port=2
  TRUE ROLL : Inport  Port=3
  ESTIMATED ROLL : Inport  Port=4
  TRUE YAW : Inport  Port=5
  ESTIMATED YAW : Inport  Port=6
  TRUE ALTITUDE : Inport  Port=7
  ESTIMATED ALTITUDE : Inport  Port=8
  TRUE AIRSPEED : Inport  Port=9
  ESTIMATED AIRSPEED : Inport  Port=10
  AIRSPEED ERROR : Scope
  ALTITUDE ERROR : Scope
  Display{,1..4} (5 alike) : Display
  PITCH ERROR : Scope
  ROLL ERROR : Scope
  Sum{,1..4} (5 alike) : Sum  Inputs=|+-
  To Workspace : ToWorkspace  VariableName=pitch_error  SampleTime=-1
  To Workspace1 : ToWorkspace  VariableName=roll_error  SampleTime=-1
  To Workspace2 : ToWorkspace  VariableName=yaw_error  SampleTime=-1
  To Workspace3 : ToWorkspace  VariableName=altitude_error  SampleTime=-1
  To Workspace4 : ToWorkspace  VariableName=airspeed_error  SampleTime=-1
  YAW ERROR : Scope
  wires:
  TRUE PITCH/1 -> Sum/1
  ESTIMATED PITCH/1 -> Sum/2
  TRUE ROLL/1 -> Sum1/1
  ESTIMATED ROLL/1 -> Sum1/2
  TRUE YAW/1 -> Sum2/1
  ESTIMATED YAW/1 -> Sum2/2
  TRUE ALTITUDE/1 -> Sum3/1
  ESTIMATED ALTITUDE/1 -> Sum3/2
  TRUE AIRSPEED/1 -> Sum4/1
  ESTIMATED AIRSPEED/1 -> Sum4/2
  Sum/1 -> To Workspace/1, Display/1, PITCH ERROR/1
  Sum1/1 -> To Workspace1/1, Display1/1, ROLL ERROR/1
  Sum2/1 -> To Workspace2/1, Display2/1, YAW ERROR/1
  Sum3/1 -> To Workspace3/1, Display3/1, ALTITUDE ERROR/1
  Sum4/1 -> To Workspace4/1, Display4/1, AIRSPEED ERROR/1

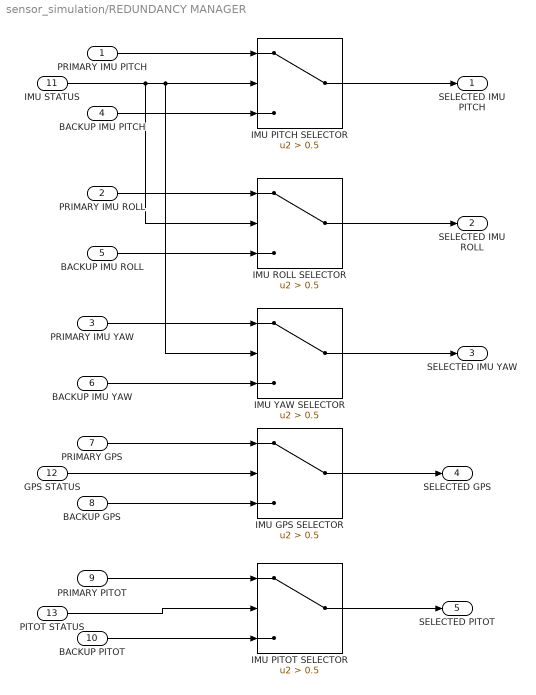
== system sensor_simulation/REDUNDANCY MANAGER ==
  PRIMARY IMU PITCH : Inport
  PRIMARY IMU ROLL : Inport  Port=2
  PRIMARY IMU YAW : Inport  Port=3
  BACKUP IMU PITCH : Inport  Port=4
  BACKUP IMU ROLL : Inport  Port=5
  BACKUP IMU YAW : Inport  Port=6
  PRIMARY GPS : Inport  Port=7
  BACKUP GPS : Inport  Port=8
  PRIMARY PITOT : Inport  Port=9
  BACKUP PITOT : Inport  Port=10
  IMU STATUS : Inport  Port=11
  GPS STATUS : Inport  Port=12
  PITOT STATUS : Inport  Port=13
  IMU GPS SELECTOR : Switch  Criteria=u2 > Threshold  Threshold=0.5
  IMU PITCH SELECTOR : Switch  Criteria=u2 > Threshold  Threshold=0.5
  IMU PITOT SELECTOR : Switch  Criteria=u2 > Threshold  Threshold=0.5
  IMU ROLL SELECTOR : Switch  Criteria=u2 > Threshold  Threshold=0.5
  IMU YAW SELECTOR : Switch  Criteria=u2 > Threshold  Threshold=0.5
  SELECTED IMU PITCH : Outport
  SELECTED IMU ROLL : Outport  Port=2
  SELECTED IMU YAW : Outport  Port=3
  SELECTED GPS : Outport  Port=4
  SELECTED PITOT : Outport  Port=5
  wires:
  PRIMARY IMU PITCH/1 -> IMU PITCH SELECTOR/1
  IMU STATUS/1 -> IMU ROLL SELECTOR/2, IMU YAW SELECTOR/2, IMU PITCH SELECTOR/2
  BACKUP IMU PITCH/1 -> IMU PITCH SELECTOR/3
  IMU PITCH SELECTOR/1 -> SELECTED IMU PITCH/1
  PRIMARY IMU ROLL/1 -> IMU ROLL SELECTOR/1
  BACKUP IMU ROLL/1 -> IMU ROLL SELECTOR/3
  IMU ROLL SELECTOR/1 -> SELECTED IMU ROLL/1
  PRIMARY IMU YAW/1 -> IMU YAW SELECTOR/1
  BACKUP IMU YAW/1 -> IMU YAW SELECTOR/3
  PRIMARY GPS/1 -> IMU GPS SELECTOR/1
  BACKUP GPS/1 -> IMU GPS SELECTOR/3
  IMU YAW SELECTOR/1 -> SELECTED IMU YAW/1
  IMU GPS SELECTOR/1 -> SELECTED GPS/1
  PRIMARY PITOT/1 -> IMU PITOT SELECTOR/1
  BACKUP PITOT/1 -> IMU PITOT SELECTOR/3
  IMU PITOT SELECTOR/1 -> SELECTED PITOT/1
  GPS STATUS/1 -> IMU GPS SELECTOR/2
  PITOT STATUS/1 -> IMU PITOT SELECTOR/2

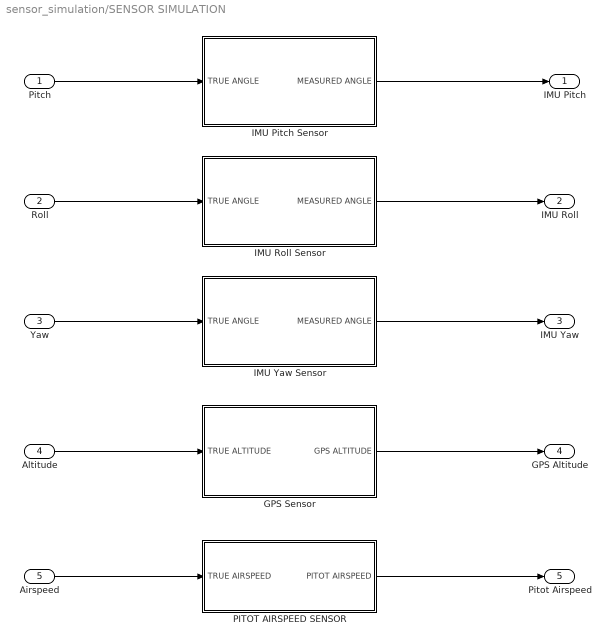
== system sensor_simulation/SENSOR SIMULATION ==
  Pitch : Inport
  Roll : Inport  Port=2
  Yaw : Inport  Port=3
  Altitude : Inport  Port=4
  Airspeed : Inport  Port=5
  " GPS Sensor" : Subsystem
  " IMU Pitch Sensor " : Subsystem
  " IMU Roll Sensor" : Subsystem
  " IMU Yaw Sensor" : Subsystem
  PITOT AIRSPEED SENSOR : Subsystem
  IMU Pitch : Outport
  IMU Roll : Outport  Port=2
  IMU Yaw : Outport  Port=3
  GPS Altitude : Outport  Port=4
  Pitot Airspeed : Outport  Port=5
  wires:
  Pitch/1 -> " IMU Pitch Sensor "/1(TRUE ANGLE)
  " IMU Pitch Sensor "/1(MEASURED ANGLE) -> IMU Pitch/1
  Roll/1 -> " IMU Roll Sensor"/1(TRUE ANGLE)
  Yaw/1 -> " IMU Yaw Sensor"/1(TRUE ANGLE)
  " IMU Roll Sensor"/1(MEASURED ANGLE) -> IMU Roll/1
  " IMU Yaw Sensor"/1(MEASURED ANGLE) -> IMU Yaw/1
  Altitude/1 -> " GPS Sensor"/1(TRUE ALTITUDE)
  " GPS Sensor"/1(GPS ALTITUDE) -> GPS Altitude/1
  Airspeed/1 -> PITOT AIRSPEED SENSOR/1(TRUE AIRSPEED)
  PITOT AIRSPEED SENSOR/1(PITOT AIRSPEED) -> Pitot Airspeed/1

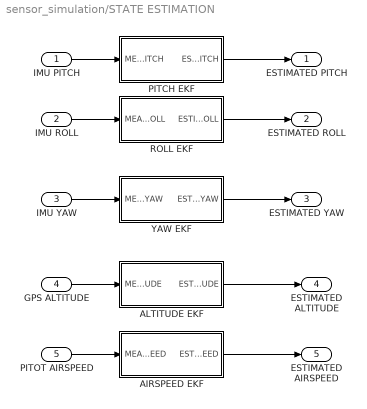
== system sensor_simulation/STATE ESTIMATION ==
  IMU PITCH : Inport
  IMU ROLL : Inport  Port=2
  IMU YAW : Inport  Port=3
  GPS ALTITUDE : Inport  Port=4
  PITOT AIRSPEED : Inport  Port=5
  AIRSPEED EKF : Subsystem
  ALTITUDE EKF : Subsystem
  PITCH EKF : Subsystem
  ROLL EKF : Subsystem
  YAW EKF : Subsystem
  ESTIMATED PITCH : Outport
  ESTIMATED ROLL : Outport  Port=2
  ESTIMATED YAW : Outport  Port=3
  ESTIMATED ALTITUDE : Outport  Port=4
  ESTIMATED AIRSPEED : Outport  Port=5
  wires:
  IMU PITCH/1 -> PITCH EKF/1(MEASURED PITCH)
  PITCH EKF/1(ESTIMATED PITCH) -> ESTIMATED PITCH/1
  GPS ALTITUDE/1 -> ALTITUDE EKF/1(MEASURED ALTITUDE)
  ROLL EKF/1(ESTIMATED ROLL) -> ESTIMATED ROLL/1
  IMU ROLL/1 -> ROLL EKF/1(MEASURED ROLL)
  IMU YAW/1 -> YAW EKF/1(MEASURED YAW)
  YAW EKF/1(ESTIMATED YAW) -> ESTIMATED YAW/1
  ALTITUDE EKF/1(ESTIMATED ALTITUDE) -> ESTIMATED ALTITUDE/1
  PITOT AIRSPEED/1 -> AIRSPEED EKF/1(MEASURED AIRSPEED)
  AIRSPEED EKF/1(ESTIMATED AIRSPEED) -> ESTIMATED AIRSPEED/1

== system sensor_simulation/AIRCRAFT PLANT/AIRSPEED DYNAMICS ==
  "THROTTLE " : Inport
  Transfer Fcn : TransferFcn  Denominator=[5 1]
  AIRSPEED : Outport
  wires:
  "THROTTLE "/1 -> Transfer Fcn/1
  Transfer Fcn/1 -> AIRSPEED/1

== system sensor_simulation/AIRCRAFT PLANT/ALTITUDE DYNAMICS ==
  PITCH : Inport
  Transfer Fcn : TransferFcn  Denominator=[10 1]
  ALTITUDE : Outport
  wires:
  PITCH/1 -> Transfer Fcn/1
  Transfer Fcn/1 -> ALTITUDE/1

== system sensor_simulation/AIRCRAFT PLANT/PITCH DYNAMICS ==
  ELEVATOR : Inport
  Transfer Fcn : TransferFcn  Denominator=[3 1]
  PITCH : Outport
  wires:
  ELEVATOR/1 -> Transfer Fcn/1
  Transfer Fcn/1 -> PITCH/1

== system sensor_simulation/AIRCRAFT PLANT/ROLL DYNAMICS ==
  AILERON : Inport
  Transfer Fcn : TransferFcn  Denominator=[2 1]
  ROLL : Outport
  wires:
  AILERON/1 -> Transfer Fcn/1
  Transfer Fcn/1 -> ROLL/1

== system sensor_simulation/AIRCRAFT PLANT/YAW DYNAMICS ==
  RUDDER : Inport
  Transfer Fcn : TransferFcn  Denominator=[4 1]
  YAW : Outport
  wires:
  RUDDER/1 -> Transfer Fcn/1
  Transfer Fcn/1 -> YAW/1

== system sensor_simulation/FLIGHT MODE MANAGER/AUTOPILOT MODES ==
  CURRENT PITCH : Inport
  MODE : Inport  Port=2
  CURRENT ALTITUDE : Inport  Port=3
  TARGET ALTITUDE : Inport  Port=4
  ALTITUDE HOLD MODE : Subsystem
  PITCH HOLD MODE : Subsystem
  PITCH HOLD OUTPUT : Outport
  ALTITUDE HOLD OUTPUT : Outport  Port=2
  wires:
  PITCH HOLD MODE/1(DESIRED PITCH) -> PITCH HOLD OUTPUT/1
  CURRENT PITCH/1 -> PITCH HOLD MODE/1(CURRENT PITCH)
  MODE/1 -> PITCH HOLD MODE/2(HOLD ENABLE)
  TARGET ALTITUDE/1 -> ALTITUDE HOLD MODE/2(TARGET ALTITUDE)
  CURRENT ALTITUDE/1 -> ALTITUDE HOLD MODE/1(CURRENT ALTITUDE)
  ALTITUDE HOLD MODE/1(DESIRED PITCH) -> ALTITUDE HOLD OUTPUT/1

== system sensor_simulation/SENSOR SIMULATION/ GPS Sensor ==
  TRUE ALTITUDE : Inport
  " Bias Adder " : Sum
  " GPS bias" : Constant  Value=0.02
  " Noise Adder" : Sum
  GPS Delay : TransportDelay  DelayTime=0.2
  GPS Noise : simulink/Sources/Band-Limited White Noise  Cov=1e-5  Ts=0.1  seed=45678
  GPS ALTITUDE : Outport
  wires:
  TRUE ALTITUDE/1 -> GPS Delay/1
  GPS Noise/1 -> " Noise Adder"/1
  GPS Delay/1 -> " Noise Adder"/2
  " Noise Adder"/1 -> " Bias Adder "/1
  " GPS bias"/1 -> " Bias Adder "/2
  " Bias Adder "/1 -> GPS ALTITUDE/1

== system sensor_simulation/SENSOR SIMULATION/ IMU Pitch Sensor  ==
  TRUE ANGLE : Inport
  " Bias Adder" : Sum
  " Noise Adder" : Sum
  " Bias" : Constant  Value=0.005
  Measurement Noise : simulink/Sources/Band-Limited White Noise  Cov=1e-6  Ts=0.01  seed=12345
  MEASURED ANGLE : Outport
  wires:
  " Bias Adder"/1 -> MEASURED ANGLE/1
  Measurement Noise/1 -> " Noise Adder"/1
  " Noise Adder"/1 -> " Bias Adder"/2
  " Bias"/1 -> " Bias Adder"/1
  TRUE ANGLE/1 -> " Noise Adder"/2

== system sensor_simulation/SENSOR SIMULATION/ IMU Roll Sensor ==
  TRUE ANGLE : Inport
  " Pitch Bias Adder" : Sum
  " Pitch Noise Adder" : Sum
  Pitch Noise : simulink/Sources/Band-Limited White Noise  Cov=1e-6  Ts=0.01  seed=23456
  Pitch bias : Constant  Value=0.005
  MEASURED ANGLE : Outport
  wires:
  " Pitch Bias Adder"/1 -> MEASURED ANGLE/1
  Pitch Noise/1 -> " Pitch Noise Adder"/1
  " Pitch Noise Adder"/1 -> " Pitch Bias Adder"/2
  Pitch bias/1 -> " Pitch Bias Adder"/1
  TRUE ANGLE/1 -> " Pitch Noise Adder"/2

== system sensor_simulation/SENSOR SIMULATION/ IMU Yaw Sensor ==
  TRUE ANGLE : Inport
  " Pitch Bias Adder" : Sum
  " Pitch Noise Adder" : Sum
  Pitch Noise : simulink/Sources/Band-Limited White Noise  Cov=1e-6  Ts=0.01  seed=34567
  Pitch bias : Constant  Value=0.005
  MEASURED ANGLE : Outport
  wires:
  " Pitch Bias Adder"/1 -> MEASURED ANGLE/1
  Pitch Noise/1 -> " Pitch Noise Adder"/1
  " Pitch Noise Adder"/1 -> " Pitch Bias Adder"/2
  Pitch bias/1 -> " Pitch Bias Adder"/1
  TRUE ANGLE/1 -> " Pitch Noise Adder"/2

== system sensor_simulation/SENSOR SIMULATION/PITOT AIRSPEED SENSOR ==
  TRUE AIRSPEED : Inport
  " Bias Adder" : Sum
  " Noise Adder" : Sum
  " Bias" : Constant  Value=0.02
  Measurement Noise : simulink/Sources/Band-Limited White Noise  Cov=1e-6  Ts=0.01  seed=12345
  PITOT AIRSPEED : Outport
  wires:
  " Noise Adder"/1 -> " Bias Adder"/2
  TRUE AIRSPEED/1 -> " Noise Adder"/2
  " Bias"/1 -> " Bias Adder"/1
  " Bias Adder"/1 -> PITOT AIRSPEED/1
  Measurement Noise/1 -> " Noise Adder"/1

== system sensor_simulation/STATE ESTIMATION/AIRSPEED EKF ==
  MEASURED AIRSPEED : Inport
  CORRECTION STEP : Subsystem
  COVARIANCE MEMORY : UnitDelay  InitialCondition=1  SampleTime=-1
  MEASUREMENT NOISE(R) : Constant  Value=0.01
  PREDICTION STEP : Subsystem
  STATE MEMORY : UnitDelay  SampleTime=-1
  ESTIMATED AIRSPEED : Outport
  wires:
  MEASURED AIRSPEED/1 -> CORRECTION STEP/3(MEASURED AIRSPEED)
  STATE MEMORY/1 -> PREDICTION STEP/1(PREVIOUS STATE)
  PREDICTION STEP/2(PREDICTED COVARIANCE) -> CORRECTION STEP/2(PREDICTED COVARIANCE)
  COVARIANCE MEMORY/1 -> PREDICTION STEP/2(PREVIOUS COVARIANCE)
  CORRECTION STEP/2(UPDATED COVARIANCE) -> COVARIANCE MEMORY/1
  PREDICTION STEP/1(PREDICTED STATE) -> CORRECTION STEP/1(PREDICTED STATE)
  MEASUREMENT NOISE(R)/1 -> CORRECTION STEP/4(MEASUREMENT COVARIANCE)
  CORRECTION STEP/1(UPDATED STATE) -> ESTIMATED AIRSPEED/1, STATE MEMORY/1

== system sensor_simulation/STATE ESTIMATION/ALTITUDE EKF ==
  MEASURED ALTITUDE : Inport
  CORRECTION STEP : Subsystem
  COVARIANCE MEMORY : UnitDelay  InitialCondition=1  SampleTime=-1
  MEASUREMENT NOISE(R) : Constant  Value=0.01
  PREDICTION STEP : Subsystem
  STATE MEMORY : UnitDelay  SampleTime=-1
  ESTIMATED ALTITUDE : Outport
  wires:
  MEASURED ALTITUDE/1 -> CORRECTION STEP/3(MEASURED ALTITUDE)
  STATE MEMORY/1 -> PREDICTION STEP/1(PREVIOUS STATE)
  PREDICTION STEP/2(PREDICTED COVARIANCE) -> CORRECTION STEP/2(PREDICTED COVARIANCE)
  COVARIANCE MEMORY/1 -> PREDICTION STEP/2(PREVIOUS COVARIANCE)
  CORRECTION STEP/2(UPDATED COVARIANCE) -> COVARIANCE MEMORY/1
  PREDICTION STEP/1(PREDICTED STATE) -> CORRECTION STEP/1(PREDICTED STATE)
  MEASUREMENT NOISE(R)/1 -> CORRECTION STEP/4(MEASUREMENT COVARIANCE)
  CORRECTION STEP/1(UPDATED STATE) -> ESTIMATED ALTITUDE/1, STATE MEMORY/1

== system sensor_simulation/STATE ESTIMATION/PITCH EKF ==
  MEASURED PITCH : Inport
  CORRECTION STEP : Subsystem
  COVARIANCE MEMORY : UnitDelay  InitialCondition=1  SampleTime=-1
  MEASUREMENT NOISE(R) : Constant  Value=0.01
  PREDICTION STEP : Subsystem
  STATE MEMORY : UnitDelay  SampleTime=-1
  ESTIMATED PITCH : Outport
  wires:
  STATE MEMORY/1 -> PREDICTION STEP/1(PREVIOUS STATE)
  COVARIANCE MEMORY/1 -> PREDICTION STEP/2(PREVIOUS COVARIANCE)
  CORRECTION STEP/2(UPDATED COVARIANCE) -> COVARIANCE MEMORY/1
  MEASUREMENT NOISE(R)/1 -> CORRECTION STEP/4(MEASUREMENT COVARIANCE)
  PREDICTION STEP/1(PREDICTED STATE) -> CORRECTION STEP/1(PREDICTED STATE)
  PREDICTION STEP/2(PREDICTED COVARIANCE) -> CORRECTION STEP/2(PREDICTED COVARIANCE)
  MEASURED PITCH/1 -> CORRECTION STEP/3(MEASURED PITCH)
  CORRECTION STEP/1(UPDATED STATE) -> ESTIMATED PITCH/1, STATE MEMORY/1

== system sensor_simulation/STATE ESTIMATION/ROLL EKF ==
  MEASURED ROLL : Inport
  CORRECTION STEP : Subsystem
  COVARIANCE MEMORY : UnitDelay  InitialCondition=1  SampleTime=-1
  MEASUREMENT NOISE(R) : Constant  Value=0.01
  PREDICTION STEP : Subsystem
  STATE MEMORY : UnitDelay  SampleTime=-1
  ESTIMATED ROLL : Outport
  wires:
  PREDICTION STEP/2(PREDICTED COVARIANCE) -> CORRECTION STEP/2(PREDICTED COVARIANCE)
  COVARIANCE MEMORY/1 -> PREDICTION STEP/2(PREVIOUS COVARIANCE)
  CORRECTION STEP/2(UPDATED COVARIANCE) -> COVARIANCE MEMORY/1
  PREDICTION STEP/1(PREDICTED STATE) -> CORRECTION STEP/1(PREDICTED STATE)
  STATE MEMORY/1 -> PREDICTION STEP/1(PREVIOUS STATE)
  MEASURED ROLL/1 -> CORRECTION STEP/3(MEASURED ROLL)
  CORRECTION STEP/1(UPDATED STATE) -> ESTIMATED ROLL/1, STATE MEMORY/1
  MEASUREMENT NOISE(R)/1 -> CORRECTION STEP/4(MEASUREMENT COVARIANCE)

== system sensor_simulation/STATE ESTIMATION/YAW EKF ==
  MEASURED YAW : Inport
  CORRECTION STEP : Subsystem
  COVARIANCE MEMORY : UnitDelay  InitialCondition=1  SampleTime=-1
  MEASUREMENT NOISE(R) : Constant  Value=0.01
  PREDICTION STEP : Subsystem
  STATE MEMORY : UnitDelay  SampleTime=-1
  ESTIMATED YAW : Outport
  wires:
  PREDICTION STEP/2(PREDICTED COVARIANCE) -> CORRECTION STEP/2(PREDICTED COVARIANCE)
  COVARIANCE MEMORY/1 -> PREDICTION STEP/2(PREVIOUS COVARIANCE)
  CORRECTION STEP/2(UPDATED COVARIANCE) -> COVARIANCE MEMORY/1
  PREDICTION STEP/1(PREDICTED STATE) -> CORRECTION STEP/1(PREDICTED STATE)
  STATE MEMORY/1 -> PREDICTION STEP/1(PREVIOUS STATE)
  MEASURED YAW/1 -> CORRECTION STEP/3(MEASURED YAW)
  CORRECTION STEP/1(UPDATED STATE) -> ESTIMATED YAW/1, STATE MEMORY/1
  MEASUREMENT NOISE(R)/1 -> CORRECTION STEP/4(MEASUREMENT COVARIANCE)

== system sensor_simulation/FLIGHT MODE MANAGER/AUTOPILOT MODES/ALTITUDE HOLD MODE ==
  CURRENT ALTITUDE : Inport
  TARGET ALTITUDE : Inport  Port=2
  " ALTITUDE ERROR" : Sum  Inputs=+-
  ALTITUDE PID : simulink/Continuous/PID Controller  Controller=PID  TimeDomain=Continuous-time  SampleTime=-1  IntegratorMethod=Forward Euler  FilterMethod=Forward Euler  Form=Parallel  UseFilter=on  ControllerParametersSource=internal  P=1  I=1  D=0  N=100  InitialConditionSource=internal  InitialConditionForIntegrator=0  InitialConditionForFilter=0  ExternalReset=none  LimitOutput=off  UpperSaturationLimit=inf  LowerSaturationLimit=-inf  LinearizeAsGain=on  AntiWindupMode=none  Kb=1  TrackingMode=off  Kt=1  PParamMin=[]  PParamMax=[]  IParamMin=[]  IParamMax=[]  DParamMin=[]  DParamMax=[]  NParamMin=[]  NParamMax=[]  KbParamMin=[]  KbParamMax=[]  KtParamMin=[]  KtParamMax=[]  POutMin=[]  POutMax=[]  IOutMin=[]  IOutMax=[]  DOutMin=[]  DOutMax=[]  NOutMin=[]  NOutMax=[]  KbOutMin=[]  KbOutMax=[]  KtOutMin=[]  KtOutMax=[]  IntegratorOutMin=[]  IntegratorOutMax=[]  FilterOutMin=[]  FilterOutMax=[]  SumOutMin=[]  SumOutMax=[]  SumI1OutMin=[]  SumI1OutMax=[]  SumI2OutMin=[]  SumI2OutMax=[]  SumI3OutMin=[]  SumI3OutMax=[]  SumDOutMin=[]  SumDOutMax=[]  SaturationOutMin=[]  SaturationOutMax=[]  IntegratorContinuousStateAttributes=''  IntegratorStateMustResolveToSignalObject=off  IntegratorRTWStateStorageClass=Auto  FilterContinuousStateAttributes=''  FilterStateMustResolveToSignalObject=off  FilterRTWStateStorageClass=Auto  DifferentiatorICPrevScaledInput=0  DifferentiatorOutMin=[]  DifferentiatorOutMax=[]  FilterDiffOutCoefMin=[]  FilterDiffOutCoefMax=[]  SumDenOutMin=[]  SumDenOutMax=[]  SumNumOutMin=[]  SumNumOutMax=[]  ReciprocalOutMin=[]  ReciprocalOutMax=[]  DivideOutMin=[]  DivideOutMax=[]  TunerSelectOption=Transfer Function Based (PID Tuner App)
  PITCH LIMIT : Saturate  UpperLimit=15  LowerLimit=-15
  DESIRED PITCH : Outport
  wires:
  TARGET ALTITUDE/1 -> " ALTITUDE ERROR"/1
  CURRENT ALTITUDE/1 -> " ALTITUDE ERROR"/2
  ALTITUDE PID/1 -> PITCH LIMIT/1
  PITCH LIMIT/1 -> DESIRED PITCH/1
  " ALTITUDE ERROR"/1 -> ALTITUDE PID/1

== system sensor_simulation/FLIGHT MODE MANAGER/AUTOPILOT MODES/PITCH HOLD MODE ==
  CURRENT PITCH : Inport
  HOLD ENABLE : Inport  Port=2
  HOLD SWITCH : Switch  Criteria=u2 > Threshold  Threshold=0.5
  PITCH MEMORY : UnitDelay  SampleTime=-1
  DESIRED PITCH : Outport
  wires:
  CURRENT PITCH/1 -> HOLD SWITCH/1
  HOLD ENABLE/1 -> HOLD SWITCH/2
  PITCH MEMORY/1 -> HOLD SWITCH/3
  HOLD SWITCH/1 -> PITCH MEMORY/1, DESIRED PITCH/1

== system sensor_simulation/STATE ESTIMATION/AIRSPEED EKF/CORRECTION STEP ==
  PREDICTED STATE : Inport
  PREDICTED COVARIANCE : Inport  Port=2
  MEASURED AIRSPEED : Inport  Port=3
  MEASUREMENT COVARIANCE : Inport  Port=4
  EKF MEASUREMENT UPDATE : MATLAB Function  TreatAsAtomicUnit=on
  UPDATED STATE : Outport
  UPDATED COVARIANCE : Outport  Port=2
  wires:
  PREDICTED STATE/1 -> EKF MEASUREMENT UPDATE/1(predicted_state)
  PREDICTED COVARIANCE/1 -> EKF MEASUREMENT UPDATE/2(predicted_covariance)
  MEASURED AIRSPEED/1 -> EKF MEASUREMENT UPDATE/3(measured_values)
  MEASUREMENT COVARIANCE/1 -> EKF MEASUREMENT UPDATE/4(R)
  EKF MEASUREMENT UPDATE/1(updated_state) -> UPDATED STATE/1
  EKF MEASUREMENT UPDATE/2(updated_covariance) -> UPDATED COVARIANCE/1

== system sensor_simulation/STATE ESTIMATION/AIRSPEED EKF/PREDICTION STEP ==
  PREVIOUS STATE : Inport
  PREVIOUS COVARIANCE : Inport  Port=2
  A : Gain
  ADD Q : Sum
  AT : Gain
  PROCESS NOISE : Constant  Value=0.001
  STATE TRANSITION : Gain
  PREDICTED STATE : Outport
  PREDICTED COVARIANCE : Outport  Port=2
  wires:
  PREVIOUS STATE/1 -> STATE TRANSITION/1
  STATE TRANSITION/1 -> PREDICTED STATE/1
  PREVIOUS COVARIANCE/1 -> A/1
  A/1 -> AT/1
  AT/1 -> ADD Q/1
  PROCESS NOISE/1 -> ADD Q/2
  ADD Q/1 -> PREDICTED COVARIANCE/1

== system sensor_simulation/STATE ESTIMATION/ALTITUDE EKF/CORRECTION STEP ==
  PREDICTED STATE : Inport
  PREDICTED COVARIANCE : Inport  Port=2
  MEASURED ALTITUDE : Inport  Port=3
  MEASUREMENT COVARIANCE : Inport  Port=4
  EKF MEASUREMENT UPDATE : MATLAB Function  TreatAsAtomicUnit=on
  UPDATED STATE : Outport
  UPDATED COVARIANCE : Outport  Port=2
  wires:
  PREDICTED STATE/1 -> EKF MEASUREMENT UPDATE/1(predicted_state)
  PREDICTED COVARIANCE/1 -> EKF MEASUREMENT UPDATE/2(predicted_covariance)
  MEASURED ALTITUDE/1 -> EKF MEASUREMENT UPDATE/3(measured_values)
  MEASUREMENT COVARIANCE/1 -> EKF MEASUREMENT UPDATE/4(R)
  EKF MEASUREMENT UPDATE/1(updated_state) -> UPDATED STATE/1
  EKF MEASUREMENT UPDATE/2(updated_covariance) -> UPDATED COVARIANCE/1

== system sensor_simulation/STATE ESTIMATION/ALTITUDE EKF/PREDICTION STEP ==
  PREVIOUS STATE : Inport
  PREVIOUS COVARIANCE : Inport  Port=2
  A : Gain
  ADD Q : Sum
  AT : Gain
  PROCESS NOISE : Constant  Value=0.001
  STATE TRANSITION : Gain
  PREDICTED STATE : Outport
  PREDICTED COVARIANCE : Outport  Port=2
  wires:
  PREVIOUS STATE/1 -> STATE TRANSITION/1
  STATE TRANSITION/1 -> PREDICTED STATE/1
  PREVIOUS COVARIANCE/1 -> A/1
  A/1 -> AT/1
  AT/1 -> ADD Q/1
  PROCESS NOISE/1 -> ADD Q/2
  ADD Q/1 -> PREDICTED COVARIANCE/1

== system sensor_simulation/STATE ESTIMATION/PITCH EKF/CORRECTION STEP ==
  PREDICTED STATE : Inport
  PREDICTED COVARIANCE : Inport  Port=2
  MEASURED PITCH : Inport  Port=3
  MEASUREMENT COVARIANCE : Inport  Port=4
  EKF MEASUREMENT UPDATE : MATLAB Function  TreatAsAtomicUnit=on
  UPDATED STATE : Outport
  UPDATED COVARIANCE : Outport  Port=2
  wires:
  PREDICTED STATE/1 -> EKF MEASUREMENT UPDATE/1(predicted_state)
  PREDICTED COVARIANCE/1 -> EKF MEASUREMENT UPDATE/2(predicted_covariance)
  MEASURED PITCH/1 -> EKF MEASUREMENT UPDATE/3(measured_pitch)
  MEASUREMENT COVARIANCE/1 -> EKF MEASUREMENT UPDATE/4(R)
  EKF MEASUREMENT UPDATE/1(updated_state) -> UPDATED STATE/1
  EKF MEASUREMENT UPDATE/2(updated_covariance) -> UPDATED COVARIANCE/1

== system sensor_simulation/STATE ESTIMATION/PITCH EKF/PREDICTION STEP ==
  PREVIOUS STATE : Inport
  PREVIOUS COVARIANCE : Inport  Port=2
  A : Gain
  ADD Q : Sum
  AT : Gain
  PROCESS NOISE : Constant  Value=0.001
  STATE TRANSITION : Gain
  PREDICTED STATE : Outport
  PREDICTED COVARIANCE : Outport  Port=2
  wires:
  PREVIOUS STATE/1 -> STATE TRANSITION/1
  STATE TRANSITION/1 -> PREDICTED STATE/1
  PREVIOUS COVARIANCE/1 -> A/1
  A/1 -> AT/1
  AT/1 -> ADD Q/1
  PROCESS NOISE/1 -> ADD Q/2
  ADD Q/1 -> PREDICTED COVARIANCE/1
